simulink model "MagLevTbx_UsbSerialPacketReceive_Block"  (R2025b)
settings: Solver=FixedStepDiscrete  StartTime=0.0  StopTime=Inf  FixedStep=0.01  RelTol=1e-3  EnableMultiTasking=on
settings Model: ExtModeTrigDuration=2  Creator=riccardo  LastModifiedBy=riccardo
settings SolverCC: AutoInsertRateTranBlk=on
settings OptimizationCC: EnhancedBackFolding=on  PassReuseOutputArgsAs=Individual arguments  ZeroExternalMemoryAtStartup=off  ZeroInternalMemoryAtStartup=off  MaxStackSize=64  OptimizeBlockOrder=speed  DifferentSizesBufferReuse=on  OptimizationCustomize=off  EfficientTunableParamExpr=on
settings DebuggingCC: ParameterTunabilityLossMsg=error
settings HardwareCC: ProdBitPerPointer=32.0  ProdBitPerSizeT=32.0  ProdBitPerPtrDiffT=32.0  ProdLargestAtomicInteger=Long  ProdLargestAtomicFloat=Double  ProdWordSize=32.0  ProdHWDeviceType=ARM Compatible->ARM Cortex
settings SFSimCC: MATLABDynamicMemAlloc=off
settings RTWCC: SystemTargetFile=ert.tlc  HardwareBoard=Teensy 4.1 (Arduino Compatible)  TemplateMakefile=ert_default_tmf  Toolchain=Arduino ARM M7  BuildConfiguration=Faster Runs  Description=Embedded Coder
settings CodeAppCC: ForceParamTrailComments=on  IgnoreCustomStorageClasses=off  OperatorAnnotations=on  SimulinkDataObjDesc=on  SFDataObjDesc=on  InsertBlockDesc=on
settings ERTTargetCC: ExtModeTransport=3.0  ExtModeStaticAlloc=on  ExtModeAutomaticAllocSize=off  ExtModeStaticAllocSize=65536.0  ExtModeMexFile=ext_xcp  ExtModeIntrfLevel=Level2 - Open  InlinedParameterPlacement=Hierarchical  RootIOFormat=Structure reference  TargetLangStandard=C99 (ISO)  SupportContinuousTime=on  SupportVariableSizeSignals=on

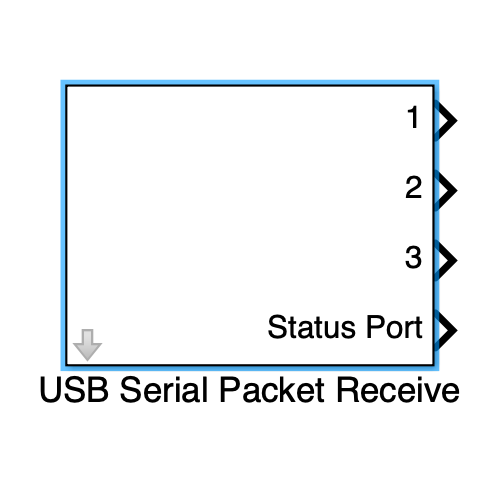
[thumbnail: Simulink's stored preview of the top-level diagram]
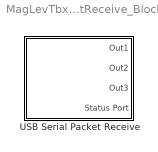
== system MagLevTbx_UsbSerialPacketReceive_Block ==
  USB Serial Packet Receive : Subsystem  mask(USB Serial Packet Receive){outputMode=HOLD Outputs, showStatusPort=on, packetSpec={'uint8', 'uint16', 'double'}, cobsEncoded=on, nullTerminated=on, sampleTime=-1, showEnablePort=off}
      mask prompts: outputMode "In case of missing packet:"; showStatusPort "Show status port"; packetSpec "Packet Specifier ( e.g. {'2*uint8', '3*single'} ):"; cobsEncoded "COBS Encoded"; nullTerminated "Null Terminated"; sampleTime "Sample time (-1 for inherited):"; showEnablePort "Show enable port"
      mask help:
      | Receive data packet from the USB serial port.
      |
      | The Status Port is set to a nonzero value when a new packet has been correctly received, and new data is available at the output ports.
      mask init:
      | cobsEncoded = logical(cobsEncoded);
      | nullTerminated = logical(nullTerminated);
      | showStatusPort = logical(showStatusPort);
      | 
      | %   init block
      | MagLevTbx_UsbSerialPacketReceive_MaskInit(gcb, packetSpec, showStatusPort, showEnablePort);
      mask Help:
      | Riccardo Antonello (riccardo.antonello@unipd.it)
      | 
      | February 18, 2026
      | 
      | Dept. of Information Engineering, University of Padova
      mask TypeOptions outputMode: HOLD Outputs | RESET Outputs
      mask Callback sampleTime: MagLevTbx_UsbSerialPacketReceive_MaskCbFcn_SampleTime();
      mask DialogControl Container3 Prompt: Communication link
      mask DialogControl Container4 Prompt: Packet definition

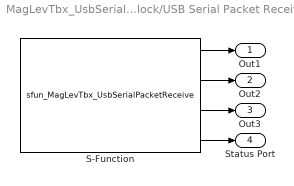
== system MagLevTbx_UsbSerialPacketReceive_Block/USB Serial Packet Receive ==
  S-Function : S-Function  FunctionName=sfun_MagLevTbx_UsbSerialPacketReceive  Parameters=packetSpec, cobsEncoded, nullTerminated, showStatusPort, outputMode, sampleTime  SFunctionDeploymentMode=off  EnableBusSupport=off
  Out1 : Outport
  Out2 : Outport  Port=2
  Out3 : Outport  Port=3
  Status Port : Outport  Port=4
  wires:
  S-Function/1 -> Out1/1
  S-Function/2 -> Out2/1
  S-Function/3 -> Out3/1
  S-Function/4 -> Status Port/1
